simulink model "simulation_ROCKET"  (R2021b)
settings: Solver=VariableStepAuto  StartTime=0.0  StopTime=650  RelTol=1e-3
model workspace (MAT data in the model file):
  M0 = [262956.456 48383.96976]
  Th = [356460 23420]
  g = 0.00981
  h = 180
  mdot = [903.20832 49.35168]
  mpl = 9072
  pich = [16.5 -2.5]
  t_v = 12.0639369756
  tb = [217.7601 642.6815]
  tbtotal = 860.4416
  tv = 12.0639369756
libraries: simulink x7
settings Model: Creator=fatima mn  LastModifiedBy=fatima mn

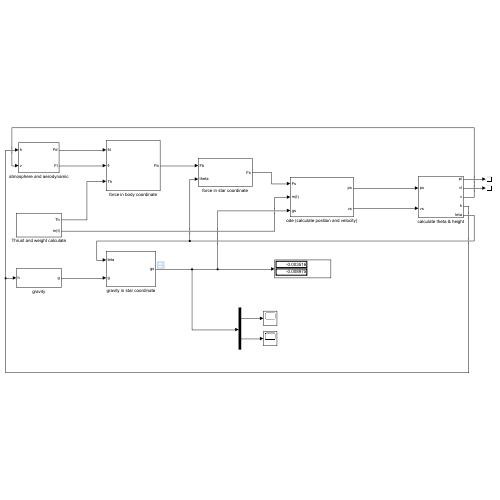
[thumbnail: Simulink's stored preview of the top-level diagram]
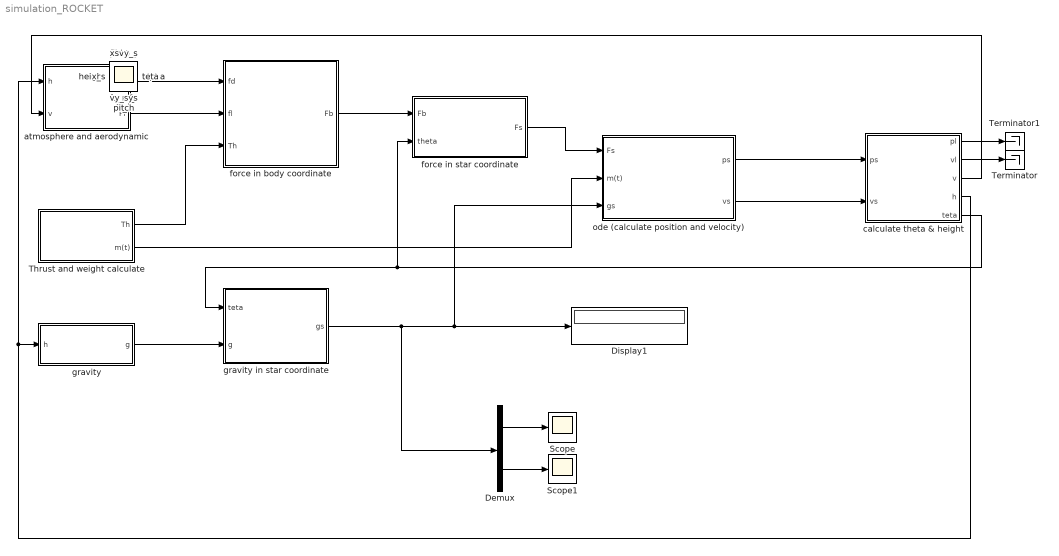
== system simulation_ROCKET ==
  Demux : Demux  Outputs=2
  Display1 : Display
  Scope : Scope
  Scope1 : Scope
  Terminator : Terminator
  Terminator1 : Terminator
  Thrust and weight calculate : Subsystem
  atmosphere and aerodynamic : Subsystem
  calculate theta & height : Subsystem
  force in body coordinate : Subsystem
  force in star coordinate : Subsystem
  gravity : Subsystem
  gravity in star coordinate : Subsystem
  ode (calculate position and velocity) : Subsystem
  M0 : Scope
  alpha : Scope
  fd : Scope
  fl : Scope
  fs_x : Scope
  fs_y : Scope
  g : Scope
  gs : Scope
  h : Scope
  height : Scope
  m_t : Scope
  phi : Scope
  pitch : Scope
  teta : Scope
  vx_s : Scope
  vy_s : Scope
  x_s : Scope
  xs : Scope
  y_s : Scope
  ys : Scope
  wires:
  gravity/1(g) -> gravity in star coordinate/2(g)
  gravity in star coordinate/1(gs) -> ode (calculate position and velocity)/3(gs), Display1/1, Demux/1
  Demux/1 -> Scope/1
  Demux/2 -> Scope1/1
  force in body coordinate/1(Fb) -> force in star coordinate/1(Fb)
  force in star coordinate/1(Fs) -> ode (calculate position and velocity)/1(Fs)
  atmosphere and aerodynamic/1(Fd) -> force in body coordinate/1(fd)
  atmosphere and aerodynamic/2(Fl) -> force in body coordinate/2(fl)
  Thrust and weight calculate/1(Th) -> force in body coordinate/3(Th)
  Thrust and weight calculate/2(m(t)) -> ode (calculate position and velocity)/2(m(t))
  ode (calculate position and velocity)/1(ps) -> calculate theta & height/1(ps)
  ode (calculate position and velocity)/2(vs) -> calculate theta & height/2(vs)
  calculate theta & height/5(teta) -> force in star coordinate/2(theta), gravity in star coordinate/1(teta)
  calculate theta & height/4(h) -> atmosphere and aerodynamic/1(h), gravity/1(h)
  calculate theta & height/3(v) -> atmosphere and aerodynamic/2(v)
  calculate theta & height/1(pl) -> Terminator1/1
  calculate theta & height/2(vl) -> Terminator/1

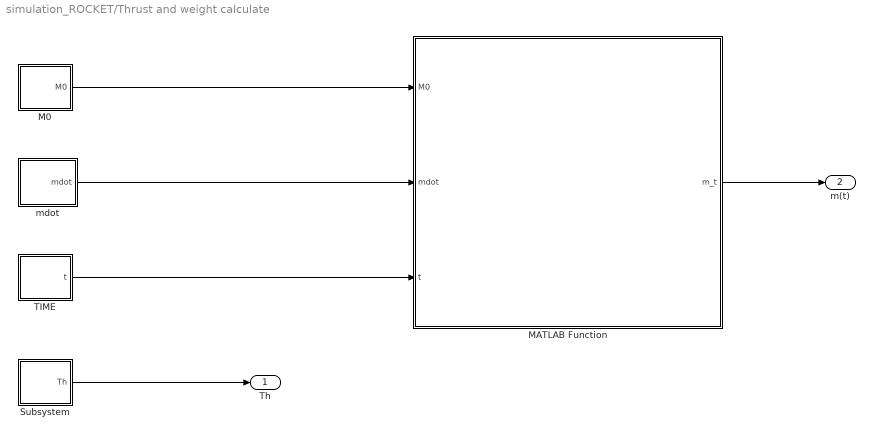
== system simulation_ROCKET/Thrust and weight calculate ==
  M0 : Subsystem
  MATLAB Function : MATLAB Function  TreatAsAtomicUnit=on
  Subsystem : Subsystem
  TIME : Subsystem
  mdot : Subsystem
  Th : Outport
  m(t) : Outport  Port=2
  wires:
  M0/1(M0) -> MATLAB Function/1(M0)
  mdot/1(mdot) -> MATLAB Function/2(mdot)
  TIME/1(t) -> MATLAB Function/3(t)
  Subsystem/1(Th) -> Th/1
  MATLAB Function/1(m_t) -> m(t)/1

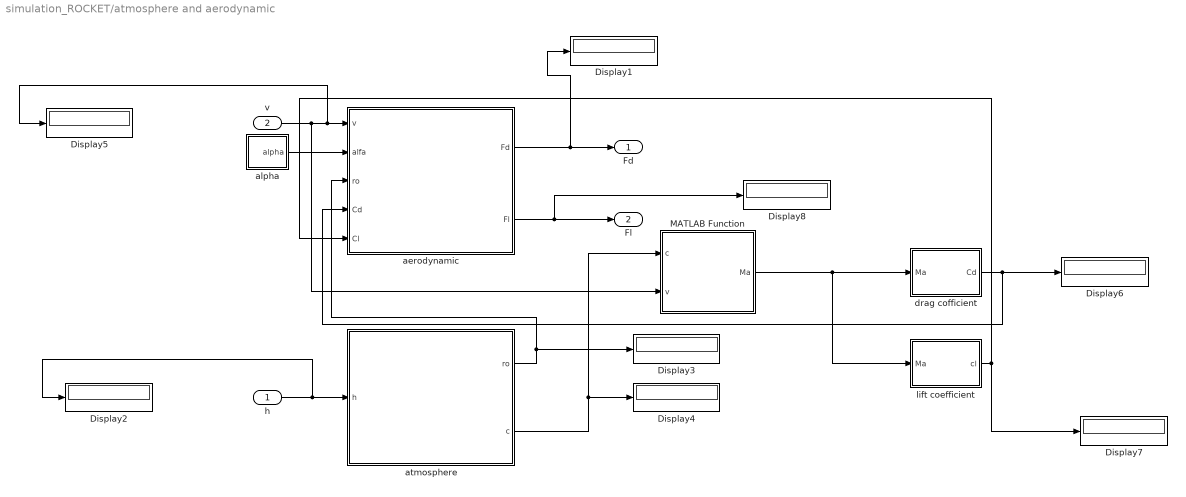
== system simulation_ROCKET/atmosphere and aerodynamic ==
  h : Inport
  v : Inport  Port=2
  Display{1..8} (8 alike) : Display
  MATLAB Function : MATLAB Function  TreatAsAtomicUnit=on
  aerodynamic : MATLAB Function  TreatAsAtomicUnit=on
  alpha : Subsystem
  atmosphere : MATLAB Function  TreatAsAtomicUnit=on
  drag cofficient : MATLAB Function  TreatAsAtomicUnit=on
  lift coefficient : MATLAB Function  TreatAsAtomicUnit=on
  Fd : Outport
  Fl : Outport  Port=2
  wires:
  alpha/1(alpha) -> aerodynamic/2(alfa)
  v/1 -> MATLAB Function/2(v), Display5/1, aerodynamic/1(v)
  h/1 -> Display2/1, atmosphere/1(h)
  atmosphere/2(c) -> Display4/1, MATLAB Function/1(c)
  atmosphere/1(ro) -> Display3/1, aerodynamic/3(ro)
  MATLAB Function/1(Ma) -> lift coefficient/1(Ma), drag cofficient/1(Ma)
  drag cofficient/1(Cd) -> aerodynamic/4(Cd), Display6/1
  lift coefficient/1(cl) -> aerodynamic/5(Cl), Display7/1
  aerodynamic/2(Fl) -> Display8/1, Fl/1
  aerodynamic/1(Fd) -> Display1/1, Fd/1

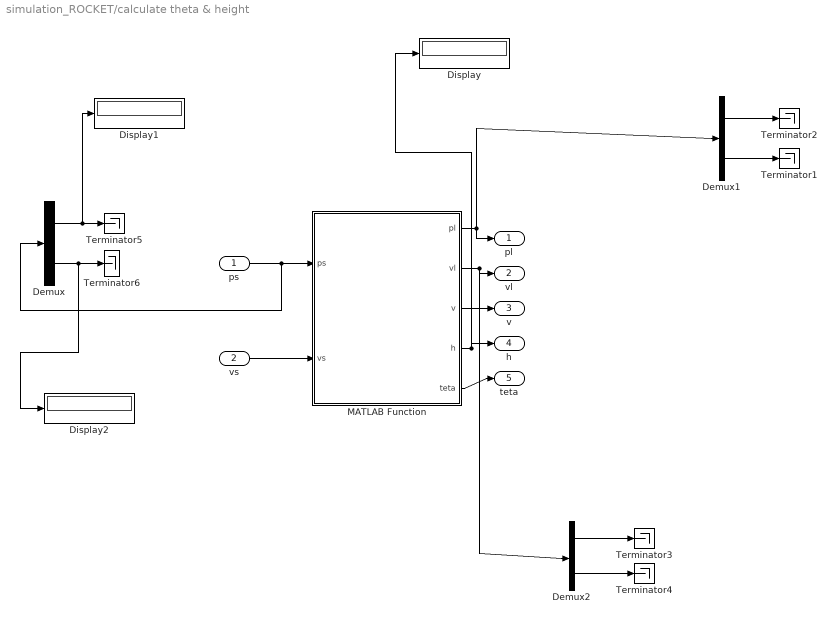
== system simulation_ROCKET/calculate theta & height ==
  ps : Inport
  vs : Inport  Port=2
  Demux : Demux  Outputs=2
  Demux1 : Demux  Outputs=2
  Demux2 : Demux  Outputs=2
  Display : Display
  Display1 : Display
  Display2 : Display
  MATLAB Function : MATLAB Function  TreatAsAtomicUnit=on
  Terminator{1..6} (6 alike) : Terminator
  pl : Outport
  vl : Outport  Port=2
  v : Outport  Port=3
  h : Outport  Port=4
  teta : Outport  Port=5
  wires:
  ps/1 -> Demux/1, MATLAB Function/1(ps)
  vs/1 -> MATLAB Function/2(vs)
  MATLAB Function/2(vl) -> Demux2/1, vl/1
  MATLAB Function/3(v) -> v/1
  MATLAB Function/1(pl) -> Demux1/1, pl/1
  MATLAB Function/4(h) -> Display/1, h/1
  MATLAB Function/5(teta) -> teta/1
  Demux1/1 -> Terminator2/1
  Demux1/2 -> Terminator1/1
  Demux2/1 -> Terminator3/1
  Demux2/2 -> Terminator4/1
  Demux/1 -> Display1/1, Terminator5/1
  Demux/2 -> Display2/1, Terminator6/1

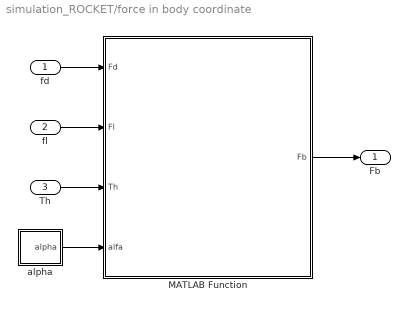
== system simulation_ROCKET/force in body coordinate ==
  fd : Inport
  fl : Inport  Port=2
  Th : Inport  Port=3
  MATLAB Function : MATLAB Function  TreatAsAtomicUnit=on
  alpha : Subsystem
  Fb : Outport
  wires:
  fd/1 -> MATLAB Function/1(Fd)
  fl/1 -> MATLAB Function/2(Fl)
  Th/1 -> MATLAB Function/3(Th)
  alpha/1(alpha) -> MATLAB Function/4(alfa)
  MATLAB Function/1(Fb) -> Fb/1

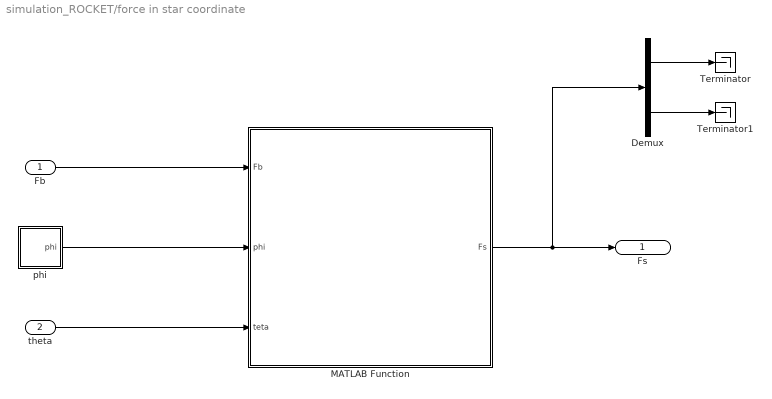
== system simulation_ROCKET/force in star coordinate ==
  Fb : Inport
  theta : Inport  Port=2
  Demux : Demux  Outputs=2
  MATLAB Function : MATLAB Function  TreatAsAtomicUnit=on
  Terminator : Terminator
  Terminator1 : Terminator
  phi : Subsystem
  Fs : Outport
  wires:
  Fb/1 -> MATLAB Function/1(Fb)
  phi/1(phi) -> MATLAB Function/2(phi)
  theta/1 -> MATLAB Function/3(teta)
  MATLAB Function/1(Fs) -> Demux/1, Fs/1
  Demux/2 -> Terminator1/1
  Demux/1 -> Terminator/1

== system simulation_ROCKET/gravity ==
  h : Inport
  MATLAB Function : MATLAB Function  TreatAsAtomicUnit=on
  g : Outport
  wires:
  h/1 -> MATLAB Function/1(h)
  MATLAB Function/1(g) -> g/1

== system simulation_ROCKET/gravity in star coordinate ==
  teta : Inport
  g : Inport  Port=2
  MATLAB Function : MATLAB Function  TreatAsAtomicUnit=on
  gs : Outport
  wires:
  teta/1 -> MATLAB Function/1(teta)
  g/1 -> MATLAB Function/2(g)
  MATLAB Function/1(gs) -> gs/1

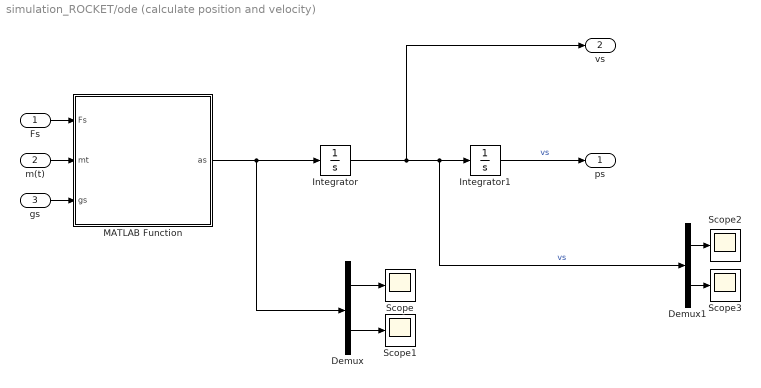
== system simulation_ROCKET/ode (calculate position and velocity) ==
  Fs : Inport
  m(t) : Inport  Port=2
  gs : Inport  Port=3
  Demux : Demux  Outputs=2
  Demux1 : Demux  Outputs=2
  Integrator : Integrator  InitialCondition=[0 ;0];
  Integrator1 : Integrator  InitialCondition=[0 ;0];
  MATLAB Function : MATLAB Function  TreatAsAtomicUnit=on
  Scope{,1..3} (4 alike) : Scope
  ps : Outport
  vs : Outport  Port=2
  wires:
  Fs/1 -> MATLAB Function/1(Fs)
  m(t)/1 -> MATLAB Function/2(mt)
  gs/1 -> MATLAB Function/3(gs)
  MATLAB Function/1(as) -> Demux/1, Integrator/1
  Integrator/1 -> vs/1, Demux1/1, Integrator1/1  "vs"
  Integrator1/1 -> ps/1  "vs"
  Demux/1 -> Scope/1
  Demux/2 -> Scope1/1
  Demux1/1 -> Scope2/1
  Demux1/2 -> Scope3/1

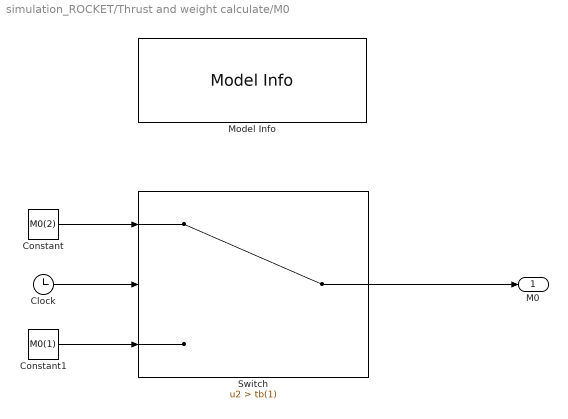
== system simulation_ROCKET/Thrust and weight calculate/M0 ==
  Clock : Clock
  Constant : Constant  Value=M0(2)
  Constant1 : Constant  Value=M0(1)
  Model Info : simulink/Model-Wide Utilities/Model Info  Frame=on  DisplayStringWithTags=total weight for each stage  HorizontalTextAlignment=Center  LeftAlignmentValue=0.5
  Switch : Switch  Criteria=u2 > Threshold  Threshold=tb(1)  ZeroCross=off
  M0 : Outport
  wires:
  Constant/1 -> Switch/1
  Constant1/1 -> Switch/3
  Clock/1 -> Switch/2
  Switch/1 -> M0/1

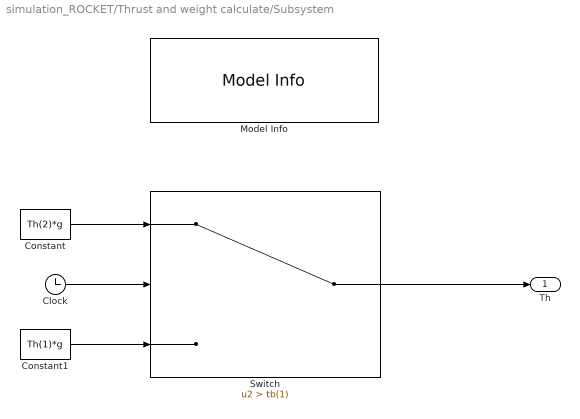
== system simulation_ROCKET/Thrust and weight calculate/Subsystem ==
  Clock : Clock
  Constant : Constant  Value=Th(2)*g
  Constant1 : Constant  Value=Th(1)*g
  Model Info : simulink/Model-Wide Utilities/Model Info  Frame=on  DisplayStringWithTags=Thrust for each stage  HorizontalTextAlignment=Center  LeftAlignmentValue=0.5
  Switch : Switch  Criteria=u2 > Threshold  Threshold=tb(1)
  Th : Outport
  wires:
  Clock/1 -> Switch/2
  Constant1/1 -> Switch/3
  Constant/1 -> Switch/1
  Switch/1 -> Th/1

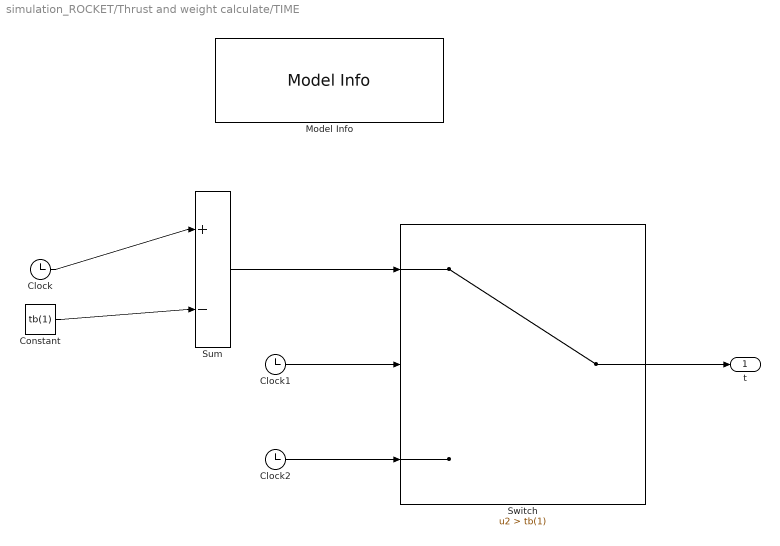
== system simulation_ROCKET/Thrust and weight calculate/TIME ==
  Clock : Clock
  Clock1 : Clock
  Clock2 : Clock
  Constant : Constant  Value=tb(1)
  Model Info : simulink/Model-Wide Utilities/Model Info  Frame=on  DisplayStringWithTags=time  HorizontalTextAlignment=Center  LeftAlignmentValue=0.5
  Sum : Sum  Inputs=|+-
  Switch : Switch  Criteria=u2 > Threshold  Threshold=tb(1)
  t : Outport
  wires:
  Clock/1 -> Sum/1
  Constant/1 -> Sum/2
  Clock2/1 -> Switch/3
  Clock1/1 -> Switch/2
  Sum/1 -> Switch/1
  Switch/1 -> t/1

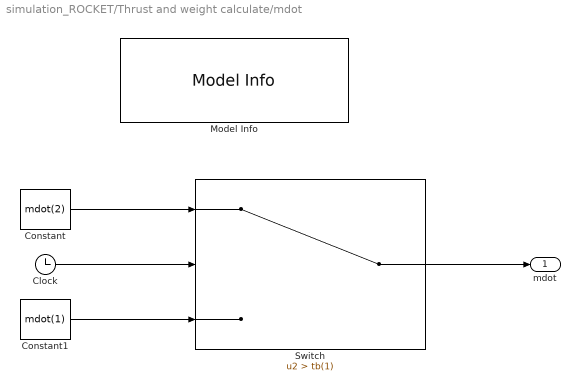
== system simulation_ROCKET/Thrust and weight calculate/mdot ==
  Clock : Clock
  Constant : Constant  Value=mdot(2)
  Constant1 : Constant  Value=mdot(1)
  Model Info : simulink/Model-Wide Utilities/Model Info  Frame=on  DisplayStringWithTags=rate of change weight each stage  HorizontalTextAlignment=Center  LeftAlignmentValue=0.5
  Switch : Switch  Criteria=u2 > Threshold  Threshold=tb(1)
  mdot : Outport
  wires:
  Clock/1 -> Switch/2
  Constant/1 -> Switch/1
  Constant1/1 -> Switch/3
  Switch/1 -> mdot/1

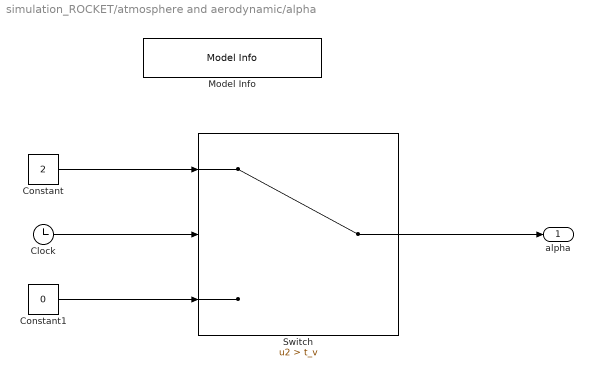
== system simulation_ROCKET/atmosphere and aerodynamic/alpha ==
  Clock : Clock
  Constant : Constant  Value=2
  Constant1 : Constant  Value=0
  Model Info : simulink/Model-Wide Utilities/Model Info  Frame=on  DisplayStringWithTags=calculate angle of attack  HorizontalTextAlignment=Center  LeftAlignmentValue=0.5
  Switch : Switch  Criteria=u2 > Threshold  Threshold=t_v
  alpha : Outport
  wires:
  Clock/1 -> Switch/2
  Constant/1 -> Switch/1
  Constant1/1 -> Switch/3
  Switch/1 -> alpha/1

== system simulation_ROCKET/force in body coordinate/alpha ==
  Clock : Clock
  Constant : Constant  Value=2
  Constant1 : Constant  Value=0
  Model Info : simulink/Model-Wide Utilities/Model Info  Frame=on  DisplayStringWithTags=calculate angle of attack  HorizontalTextAlignment=Center  LeftAlignmentValue=0.5
  Switch : Switch  Criteria=u2 > Threshold  Threshold=t_v
  alpha : Outport
  wires:
  Clock/1 -> Switch/2
  Constant/1 -> Switch/1
  Constant1/1 -> Switch/3
  Switch/1 -> alpha/1

== system simulation_ROCKET/force in star coordinate/phi ==
  MATLAB Function : MATLAB Function  TreatAsAtomicUnit=on
  alpha : Subsystem
  pitch : Subsystem
  phi : Outport
  wires:
  alpha/1(alpha) -> MATLAB Function/1(alfa)
  pitch/1(pitch) -> MATLAB Function/2(pitch)
  MATLAB Function/1(phi) -> phi/1

== system simulation_ROCKET/force in star coordinate/phi/alpha ==
  Clock : Clock
  Constant : Constant  Value=2
  Constant1 : Constant  Value=0
  Model Info : simulink/Model-Wide Utilities/Model Info  Frame=on  DisplayStringWithTags=calculate angle of attack  HorizontalTextAlignment=Center  LeftAlignmentValue=0.5
  Switch : Switch  Criteria=u2 > Threshold  Threshold=t_v
  alpha : Outport
  wires:
  Clock/1 -> Switch/2
  Constant/1 -> Switch/1
  Constant1/1 -> Switch/3
  Switch/1 -> alpha/1

== system simulation_ROCKET/force in star coordinate/phi/pitch ==
  Clock : Clock
  Constant1 : Constant  Value=tb
  Constant2 : Constant  Value=t_v
  MATLAB Function : MATLAB Function  TreatAsAtomicUnit=on
  pich : Constant  Value=pich
  pitch : Outport
  wires:
  pich/1 -> MATLAB Function/1(pich)
  Clock/1 -> MATLAB Function/2(t)
  Constant1/1 -> MATLAB Function/3(tb)
  Constant2/1 -> MATLAB Function/4(t_v)
  MATLAB Function/1(pitch) -> pitch/1

== matlab function simulation_ROCKET/force in star coordinate/MATLAB Function ==
  data: Fb input; Fs output; phi input; teta input
function Fs = fcn(Fb,phi,teta)
    
    T_SB=[cosd(phi-teta) +sind(phi-teta);
          sind(phi-teta) -cosd(phi-teta)];
    Fs=T_SB*Fb;

end

== matlab function simulation_ROCKET/ode (calculate position and velocity)/MATLAB Function ==
  data: Fs input; as output; mt input; gs input
function as = fcn(Fs,mt,gs)
    aks=Fs/mt;
    as=aks+gs;
end

== matlab function simulation_ROCKET/atmosphere and aerodynamic/atmosphere ==
  data: h input; ro output; c output
function [ro,c]=ATMOSFER(h)
% calculation of ro density air(kg/m^3) and sound velocity(m/s)
%verces hight(m)
ro=0;
c=0;
g=9.806;mo=28.966;R=8314.34;
if (h<=0) ro=1.22;c=340;end 

if (h>=0 && h<=11000) 
   hb=0 ; lm=-0.0065;   
   pb=101325.0;rob=1.2266;tmb=287.827;
   
   tm=tmb+lm*(h-hb);
   ro=rob*(tmb/tm)^(1+g*mo/(R*lm));
   c=sqrt(1.4*R*tm/mo);
   p=pb*(tmb/tm)^(g*mo/(R*lm));
end
%------------------------------------------------
if (h>11000 && h<=25000) 
   hb=11000 ; lm=0.0;   
   pb=22589;rob=.3638;tmb=216.327;
   
   tm=tmb;
   ro=rob*exp(-g*mo*(h-hb)/(R*tm));
   c=sqrt(1.4*R*tm/mo);
   p=pb*exp(-g*mo*(h-hb)/(R*tm));
end
%------------------------------------------------
if (h>25000 && h<=60960) 
   hb=25000 ; lm=0.001033;   
   pb=2475.8;rob=0.0399;tmb=216.327;
   
   tm=tmb+lm*(h-hb);
   ro=rob*(tmb/tm)^(1+g*mo/(R*lm));
   c=sqrt(1.4*R*tm/mo);
   p=pb*(tmb/tm)^(g*mo/(R*lm));
end
%------------------------------------------------
if (h>=60960 && h<=76200) 
   hb=60960 ; lm=-0.003739;   
   pb=13.1121;rob=1.8035e-4;tmb=253.4737;
   
   tm=tmb+lm*(h-hb);
   ro=rob*(tmb/tm)^(1+g*mo/(R*lm));
   c=sqrt(1.4*R*tm/mo);
   p=pb*(tmb/tm)^(g*mo/(R*lm));
end
%------------------------------------------------
if (h>76200 && h<=91440) 
   hb=76200 ; lm=0.0;   
   pb=1.2801;rob=2.2712e-5;tmb=196.4913;
   
   tm=tmb;
   ro=rob*exp(-g*mo*(h-hb)/(R*tm));
   c=sqrt(1.4*R*tm/mo);
   p=pb*exp(-g*mo*(h-hb)/(R*tm));
end
%------------------------------------------------
if (h>91440) 
   hb=91440 ; lm=0.003531;   
   pb=0.0905;rob=1.6051e-6;tmb=196.4913;
   
   tm=tmb+lm*(h-hb);
   ro=rob*(tmb/tm)^(1+g*mo/(R*lm));
   c=sqrt(1.4*R*tm/mo);
   p=pb*(tmb/tm)^(g*mo/(R*lm));
end
%------------------------------------------------

% 
% yy(1)=ro;
% yy(2)=c;

== matlab function simulation_ROCKET/calculate theta & height/MATLAB Function ==
  data: ps input; pl output; vs input; vl output; v output; h output; teta output
function [pl,vl,v,h,teta] = fcn(ps,vs)
    Re=6378;
    teta=atand(ps(1)/(Re+ps(2)));
    h=(sqrt((ps(2)+Re)^2+(ps(1)^2))-Re);
    T_LS=[cosd(teta) -sind(teta);
          sind(teta)  cosd(teta)];
    pl=T_LS*ps;
    vl=T_LS*vs;
    v=norm(vs);
end

== matlab function simulation_ROCKET/atmosphere and aerodynamic/aerodynamic ==
  data: v input; Fd output; alfa input; ro input; Cd input; Cl input; Fl output
function  [Fd,Fl]   =  faero(v,alfa,ro,Cd,Cl)
%  Calculate  aerodynamic forces(N)
    s=pi*(2.4/2)^2;
    Fd = 0.5*ro*v^2*s*Cd;
    Fl=0.5*ro*v^2*s*Cl*deg2rad(alfa);
end

== matlab function simulation_ROCKET/atmosphere and aerodynamic/MATLAB Function ==
  data: c input; Ma output; v input
function Ma = fcn(c,v)

    Ma=v/c;
end

== matlab function simulation_ROCKET/atmosphere and aerodynamic/drag cofficient ==
  data: Ma input; Cd output
function Cd = fcn(Ma)

Mac= [1.00E-01, 1.50E-01, 2.00E-01, 2.50E-01, 3.00E-01, 3.50E-01, 4.00E-01, 4.50E-01, 5.00E-01, 5.50E-01, 6.00E-01, 6.50E-01, 7.00E-01, 7.50E-01, 8.00E-01, 8.50E-01, 9.00E-01, 9.50E-01, 1.00E+00, 1.05E+00, 1.10E+00, 1.15E+00, 1.20E+00, 1.30E+00, 1.67E+00, 2.04E+00, 2.41E+00, 2.78E+00, 3.15E+00, 3.52E+00, 3.89E+00, 4.26E+00, 4.63E+00, 5.00E+00, 6.00E+00, 7.00E+00, 8.00E+00, 9.00E+00, 1.00E+01, 1.10E+01, 1.20E+01, 1.30E+01, 1.40E+01, 1.50E+01];
CD = [1.98457E-01, 1.92229E-01, 1.88068E-01, 1.84961E-01, 1.82485E-01, 1.80425E-01, 1.78661E-01, 1.77119E-01, 1.75752E-01, 1.74302E-01, 1.75826E-01, 1.90017E-01, 2.15490E-01, 2.50139E-01, 2.91750E-01, 3.51389E-01, 4.13845E-01, 4.92505E-01, 5.63296E-01, 6.31094E-01, 6.64121E-01, 6.89246E-01, 7.06884E-01, 7.35228E-01, 8.38186E-01, 7.90632E-01, 6.88748E-01, 6.60590E-01, 6.35009E-01, 6.13229E-01, 5.89903E-01, 5.69896E-01, 5.52417E-01, 5.36401E-01, 5.26189E-01, 5.05627E-01, 4.88245E-01, 4.73217E-01, 4.59966E-01, 4.52839E-01, 4.47049E-01, 4.42140E-01, 4.38247E-01, 4.35021E-01];
Cd = interp1(Mac, CD, Ma, 'pchip');

end

== matlab function simulation_ROCKET/atmosphere and aerodynamic/lift coefficient ==
  data: Ma input; cl output
function cl = fcn(Ma)

Mac= [1.00E-01, 1.50E-01, 2.00E-01, 2.50E-01, 3.00E-01, 3.50E-01, 4.00E-01, 4.50E-01, 5.00E-01, 5.50E-01, 6.00E-01, 6.50E-01, 7.00E-01, 7.50E-01, 8.00E-01, 8.50E-01, 9.00E-01, 9.50E-01, 1.00E+00, 1.05E+00, 1.10E+00, 1.15E+00, 1.20E+00, 1.30E+00, 1.67E+00, 2.04E+00, 2.41E+00, 2.78E+00, 3.15E+00, 3.52E+00, 3.89E+00, 4.26E+00, 4.63E+00, 5.00E+00,  6.00E+00, 7.00E+00, 8.00E+00, 9.00E+00, 1.00E+01, 1.10E+01, 1.20E+01, 1.30E+01, 1.40E+01, 1.50E+01];
CL = [9.4040E-02, 9.1229E-02, 8.9092E-02, 8.5098E-02, 8.3589E-02, 8.3675E-02, 8.3855E-02, 8.4024E-02, 8.4182E-02, 8.3258E-02, 8.3608E-02, 8.3482E-02, 8.2936E-02, 8.2045E-02, 8.0890E-02, 8.0302E-02, 7.8686E-02, 7.7819E-02, 7.8511E-02, 7.8576E-02, 7.8445E-02, 7.6759E-02, 7.4823E-02, 1.1368E-01, 1.1561E-01, 1.0338E-01, 8.6636E-02, 7.4759E-02, 6.3637E-02, 5.3710E-02, 5.5740E-02, 5.8011E-02, 5.9813E-02, 6.1110E-02, 6.9655E-02, 7.0597E-02, 7.1349E-02, 7.1974E-02, 7.2508E-02, 7.2810E-02, 7.4934E-02, 7.5583E-02, 7.6189E-02, 7.7068E-02];
cl = interp1(Mac, CL, Ma, 'pchip');

end

== matlab function simulation_ROCKET/Thrust and weight calculate/MATLAB Function ==
  data: M0 input; m_t output; mdot input; t input
function m_t = fcn(M0,mdot,t)

m_t=M0-mdot*t;

end

== matlab function simulation_ROCKET/gravity/MATLAB Function ==
  data: h input; g output
function g = fcn(h)
    %MU(M^3/S^2)
    mu=3.9862*10^5;
    Re=6378;
    r=Re+h;
    g=mu/r^2;
end

== matlab function simulation_ROCKET/gravity in star coordinate/MATLAB Function ==
  data: teta input; gs output; g input
function gs= fcn(teta,g)
%teta=Atan(xs/Re+ys)
    gxs=-g*sind(teta);
    gys=-g*cosd(teta);
    gs=[gxs;gys];
end

== matlab function simulation_ROCKET/force in body coordinate/MATLAB Function ==
  data: Fd input; Fb output; Fl input; Th input; alfa input
function Fb = fcn(Fd,Fl,Th,alfa)
    fxb=Th-Fd*cosd(alfa)+Fl*sind(alfa);
    fyb=-Fl*cosd(alfa)-Fd*sind(alfa);
    Fb=[fxb;fyb];
end

== matlab function simulation_ROCKET/force in star coordinate/phi/pitch/MATLAB Function ==
  data: pich input; pitch output; t input; tb input; t_v input
function pitch = fcn(pich,t,tb,t_v)
pitch=0;
if t<=t_v
    pitch=90;
elseif t>t_v && t<=tb(1)
    pitch=(90-pich(1))*((tb(1)-t)/(tb(1)-t_v))^2+pich(1);
elseif t>tb(1)
%     c0=(tand(pich(1))-tand(pich(2)))/650-tb(1);
%     tanl=tand(pich(1)-c0*tb(2));
%     pitch=atand(tanl-c0*t);
    pitch=pich(1)-((pich(1)-pich(2))/(650-tb(1)))*(t-tb(1));
end
end

== matlab function simulation_ROCKET/force in star coordinate/phi/MATLAB Function ==
  data: alfa input; phi output; pitch input
function phi = fcn(alfa,pitch)
    %pitch=gamma
    %phi=alfa+pitch;
    phi=alfa+pitch;
end
